simulink model "uavR_PID_Validation"  (R2024a)
settings: Solver=ode113  StartTime=0.0  StopTime=100  FixedStep=0.01  RelTol=1e-3  EnableMultiTasking=on
values from neighbouring files (symbols this model uses):
  alate = [-0.664377411201 -330.163387746 53.2835973356 0 0 24.9999999996 0.0408233020992 -32.3114507249 0.453859073573 1 0 0 ... (36 elements, 6x6)]    [data.mat]    (also in uavck_0.3ma.mat = [-0.227087280821 0 0 -76.755540132 38.6889917334 100.9303781)
  blate = [0  0; -3.47475022598  0.138298516457; 0.0522368492882  -0.439264414469; 0  0; 0  0; 0  0]    [data.mat]    (also in uavck_0.3ma.mat = [0.000494526671357  0.00154149546586; 0  0; 0  0; -4.1487737)
  clate = [57.2957795131 0 0 0 0 0 0 57.2957795131 0 0 0 0 ... (36 elements, 6x6)]    [data.mat]    (also in uavck_0.3ma.mat = [57.2957804904 0 0 0 0 0 0 57.2957804904 0 0 0 0 ... (36 ele)
  dlate = [0  0; 0  0; 0  0; 0  0; 0  0; 0  0]    [data.mat]    (also in uavck_0.3ma.mat)
  utrim = [-0.27394440066 -2.18120400277e-14 2.66036165513e-14 36.1693692171]    [data.mat]    (also in uavck_0.3ma.mat = [3.01593434862 -3.12927644793e-17 -4.76262648152e-17 0.40338)
  ytrim = [25 2.3396530782 1.37911498271e-14 -1.7963177274e-14 -1.87974334034e-13 100.031205124 -4.04263501627e-21 1.15674010744e-20 -9.76571062923e-22 -2.660361454e-14 2.3396530782 0 ... (13 elements, 13x1)]    [data.mat]    (also in uavck_0.3ma.mat = [100.930378182 3.74826362454 -1.61286790598e-16 4.7626264815)
settings Model: Creator=Administrator  LastModifiedBy=rzxha
settings SolverCC: AlgebraicLoopSolver=TrustRegion
settings DataIOCC: SaveFormat=Array  SignalLoggingSaveFormat=ModelDataLogs  ReturnWorkspaceOutputs=off  SignalLoggingName=sigsOut
settings OptimizationCC: BooleanDataType=off  ExpressionDepthLimit=2147483647  InitFltsAndDblsToZero=on  LifeSpan=inf
settings DebuggingCC: SaveWithParameterizedLinksMsg=none  UnderspecifiedInitializationDetection=Classic  MergeDetectMultiDrivingBlocksExec=none  SignalResolutionControl=TryResolveAllWithWarning  MultiTaskDSMMsg=warning  MultiTaskCondExecSysMsg=none  FcnCallInpInsideContextMsg=warning  UnconnectedInputMsg=warning  UnconnectedOutputMsg=warning  UnconnectedLineMsg=warning  StateNameClashWarn=warning  SFUnexpectedBacktrackingDiag=warning  SFNoUnconditionalDefaultTransitionDiag=warning  ArithmeticOperatorsInVariantConditions=warning
settings HardwareCC: ProdBitPerPointer=32  ProdBitPerSizeT=32  ProdBitPerPtrDiffT=32  ProdLargestAtomicFloat=None  ProdIntDivRoundTo=Undefined  ProdEndianess=Unspecified  ProdWordSize=32  ProdHWDeviceType=32-bit Generic  TargetUnknown=on
settings ModelReferenceCC: EnableRefExpFcnMdlSchedulingChecks=on  PropagateSignalLabelsOutOfModel=off
settings SFSimCC: SimUseLocalCustomCode=off  CustomCodeUndefinedFunction=UseInterfaceOnly
settings RTWCC: RTWUseLocalCustomCode=off  GPUComputeCapability=3.5
settings CodeAppCC: StateflowObjectComments=on
settings GRTTargetCC: TargetFcnLib=ansi_tfl_tmw.mat  TargetLangStandard=C89/C90 (ANSI)  CombineOutputUpdateFcns=off  GRTInterface=on
settings ConfigComp: CovMetricSettings=dw  CovSaveCumulativeToWorkspaceVar=on  CovSaveSingleToWorkspaceVar=on  CovExternalEMLEnable=off

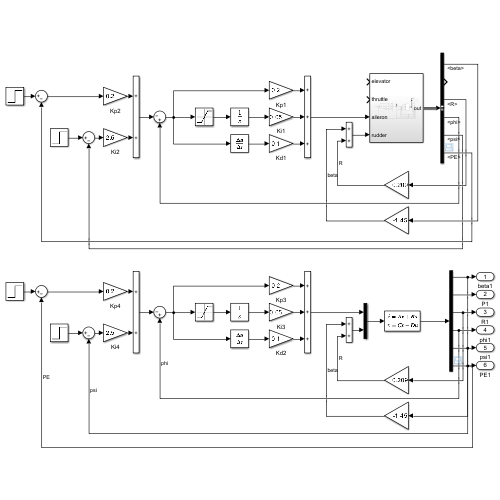
[thumbnail: Simulink's stored preview of the top-level diagram]
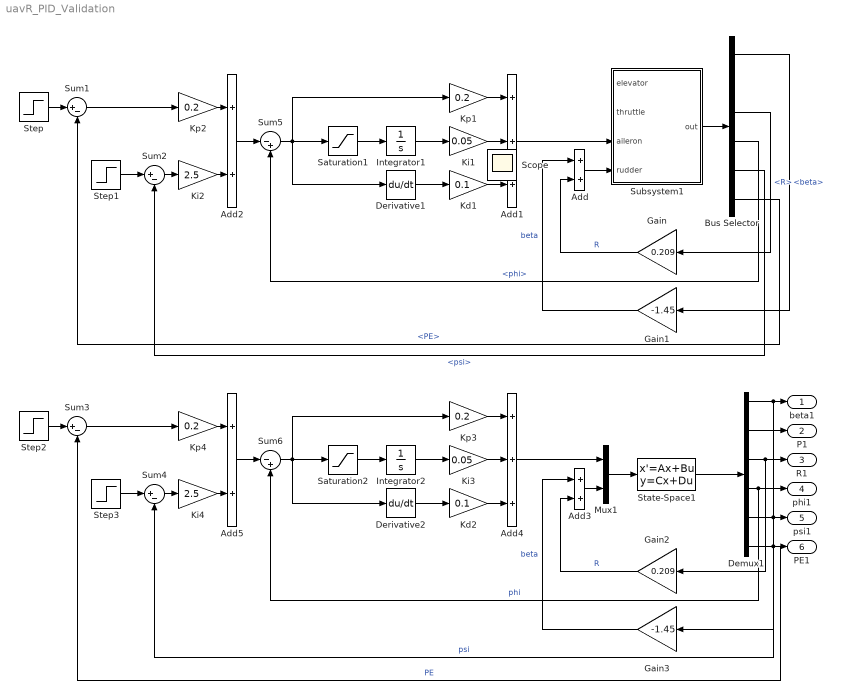
== system uavR_PID_Validation ==
  Add{,2..3,5} (4 alike) : Sum
  Add1 : Sum  Inputs=+++
  Add4 : Sum  Inputs=+++
  Bus Selector : BusSelector  OutputSignals=beta,P,R,phi,psi,PE
  Demux1 : Demux  Outputs=6
  Derivative1 : Derivative
  Derivative2 : Derivative
  Gain : Gain  Gain=0.209
  Gain1 : Gain  Gain=-1.45
  Gain2 : Gain  Gain=0.209
  Gain3 : Gain  Gain=-1.45
  Integrator1 : Integrator
  Integrator2 : Integrator
  Kd1 : Gain  Gain=0.1
  Kd2 : Gain  Gain=0.1
  Ki1 : Gain  Gain=0.05
  Ki2 : Gain  Gain=2.5
  Ki3 : Gain  Gain=0.05
  Ki4 : Gain  Gain=2.5
  Kp{1..4} (4 alike) : Gain  Gain=0.2
  Mux1 : Mux  Inputs=2
  Saturation1 : Saturate
  Saturation2 : Saturate
  State-Space1 : StateSpace  A=alate  B=blate  C=clate  D=dlate  InitialCondition=0
  Step : Step  SampleTime=0
  Step1 : Step  After=0  SampleTime=0
  Step2 : Step  SampleTime=0
  Step3 : Step  After=0  SampleTime=0
  Subsystem1 : Subsystem
  Sum{1..4} (4 alike) : Sum  Inputs=|+-
  Sum5 : Sum  Inputs=|-+
  Sum6 : Sum  Inputs=|-+
  beta1 : Outport  VectorParamsAs1DForOutWhenUnconnected=off
  P1 : Outport  Port=2  VectorParamsAs1DForOutWhenUnconnected=off
  R1 : Outport  Port=3  VectorParamsAs1DForOutWhenUnconnected=off
  phi1 : Outport  Port=4  VectorParamsAs1DForOutWhenUnconnected=off
  psi1 : Outport  Port=5  VectorParamsAs1DForOutWhenUnconnected=off
  PE1 : Outport  Port=6  VectorParamsAs1DForOutWhenUnconnected=off
  Scope : Scope
  wires:
  Subsystem1/1(out) -> Bus Selector/1
  Sum5/1 -> Saturation1/1, Kp1/1, Derivative1/1
  Step1/1 -> Sum2/1
  Kp2/1 -> Add2/1
  Sum2/1 -> Ki2/1
  Sum1/1 -> Kp2/1
  Add1/1 -> Subsystem1/3(aileron)
  Derivative1/1 -> Kd1/1
  Kd1/1 -> Add1/3
  Ki1/1 -> Add1/2
  Ki2/1 -> Add2/2
  Kp1/1 -> Add1/1
  Gain/1 -> Add/2  "R"
  Step/1 -> Sum1/1
  Add2/1 -> Sum5/1
  Saturation1/1 -> Integrator1/1
  Add/1 -> Subsystem1/4(rudder)
  Integrator1/1 -> Ki1/1
  Gain1/1 -> Add/1  "beta"
  Sum6/1 -> Saturation2/1, Kp3/1, Derivative2/1
  Step3/1 -> Sum4/1
  Kp4/1 -> Add5/1
  Sum4/1 -> Ki4/1
  Sum3/1 -> Kp4/1
  Demux1/1 -> Gain3/1, beta1/1
  Demux1/5 -> Sum4/2, psi1/1  "psi"
  Demux1/4 -> Sum6/2, phi1/1  "phi"
  Mux1/1 -> State-Space1/1
  Add4/1 -> Mux1/1
  Derivative2/1 -> Kd2/1
  Kd2/1 -> Add4/3
  Ki3/1 -> Add4/2
  Ki4/1 -> Add5/2
  Kp3/1 -> Add4/1
  Gain2/1 -> Add3/2  "R"
  Step2/1 -> Sum3/1
  Demux1/3 -> R1/1, Gain2/1
  Add5/1 -> Sum6/1
  State-Space1/1 -> Demux1/1
  Demux1/6 -> Sum3/2, PE1/1  "PE"
  Saturation2/1 -> Integrator2/1
  Demux1/2 -> P1/1
  Add3/1 -> Mux1/2
  Integrator2/1 -> Ki3/1
  Gain3/1 -> Add3/1  "beta"
  Bus Selector/1 -> Gain1/1  "<beta>"
  Bus Selector/3 -> Gain/1  "<R>"
  Bus Selector/4 -> Sum5/2  "<phi>"
  Bus Selector/6 -> Sum1/2  "<PE>"
  Bus Selector/5 -> Sum2/2  "<psi>"

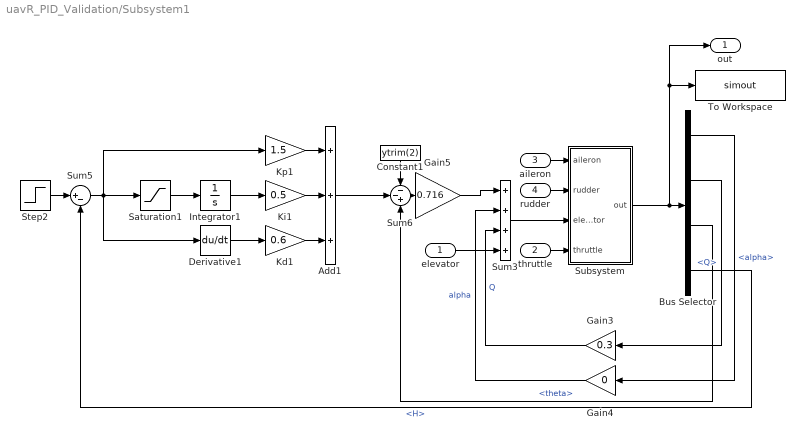
== system uavR_PID_Validation/Subsystem1 ==
  elevator : Inport
  thruttle : Inport  Port=2
  aileron : Inport  Port=3
  rudder : Inport  Port=4
  Add1 : Sum  Inputs=+++
  Bus Selector : BusSelector  OutputSignals=alpha,Q,theta,H
  Constant1 : Constant  Value=ytrim(2)
  Derivative1 : Derivative
  Gain3 : Gain  Gain=0.3
  Gain4 : Gain  Gain=0
  Gain5 : Gain  Gain=0.716
  Integrator1 : Integrator
  Kd1 : Gain  Gain=0.6
  Ki1 : Gain  Gain=0.5
  Kp1 : Gain  Gain=1.5
  Saturation1 : Saturate
  Step2 : Step  Before=1000  After=1000  SampleTime=0
  Subsystem : Subsystem
  Sum3 : Sum  Inputs=++++
  Sum5 : Sum  Inputs=|+-
  Sum6 : Sum  Inputs=--+
  To Workspace : ToWorkspace  VariableName=simout  SaveFormat=Timeseries  SampleTime=-1
  out : Outport
  wires:
  Saturation1/1 -> Integrator1/1
  Ki1/1 -> Add1/2
  Constant1/1 -> Sum6/1
  Kd1/1 -> Add1/3
  Integrator1/1 -> Ki1/1
  Kp1/1 -> Add1/1
  Gain4/1 -> Sum3/2  "alpha"
  Sum6/1 -> Gain5/1
  Derivative1/1 -> Kd1/1
  Gain3/1 -> Sum3/3  "Q"
  Bus Selector/3 -> Sum6/3  "<theta>"
  Step2/1 -> Sum5/1
  Sum5/1 -> Saturation1/1, Kp1/1, Derivative1/1
  Add1/1 -> Sum6/2
  Gain5/1 -> Sum3/1
  Subsystem/1(out) -> out/1, To Workspace/1, Bus Selector/1
  aileron/1 -> Subsystem/1(aileron)
  Bus Selector/1 -> Gain4/1  "<alpha>"
  Bus Selector/4 -> Sum5/2  "<H>"
  Bus Selector/2 -> Gain3/1  "<Q>"
  Sum3/1 -> Subsystem/3(elevator)
  rudder/1 -> Subsystem/2(rudder)
  thruttle/1 -> Subsystem/4(thruttle)
  elevator/1 -> Sum3/4

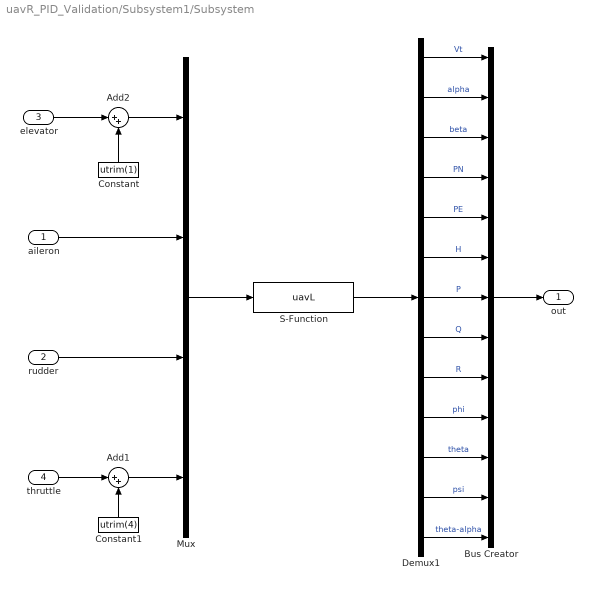
== system uavR_PID_Validation/Subsystem1/Subsystem ==
  aileron : Inport
  rudder : Inport  Port=2
  elevator : Inport  Port=3
  thruttle : Inport  Port=4
  Add1 : Sum  Inputs=|++
  Add2 : Sum  Inputs=|++
  Bus Creator : BusCreator  Inputs=13
  Constant : Constant  Value=utrim(1)
  Constant1 : Constant  Value=utrim(4)
  Demux1 : Demux  Outputs=13
  Mux : Mux
  S-Function : S-Function  FunctionName=uavL  SFunctionDeploymentMode=off  EnableBusSupport=off
  out : Outport
  wires:
  Add1/1 -> Mux/4
  thruttle/1 -> Add1/1
  Constant1/1 -> Add1/2
  rudder/1 -> Mux/3
  Demux1/4 -> Bus Creator/4  "PN"
  Add2/1 -> Mux/1
  Mux/1 -> S-Function/1
  Constant/1 -> Add2/2
  aileron/1 -> Mux/2
  elevator/1 -> Add2/1
  Demux1/11 -> Bus Creator/11  "theta"
  S-Function/1 -> Demux1/1
  Demux1/12 -> Bus Creator/12  "psi"
  Demux1/5 -> Bus Creator/5  "PE"
  Demux1/10 -> Bus Creator/10  "phi"
  Demux1/6 -> Bus Creator/6  "H"
  Demux1/2 -> Bus Creator/2  "alpha"
  Demux1/1 -> Bus Creator/1  "Vt"
  Demux1/3 -> Bus Creator/3  "beta"
  Demux1/13 -> Bus Creator/13  "theta-alpha"
  Demux1/9 -> Bus Creator/9  "R"
  Demux1/8 -> Bus Creator/8  "Q"
  Demux1/7 -> Bus Creator/7  "P"
  Bus Creator/1 -> out/1
